simulink subsystem "processor"  (R2026a)
settings: Solver=VariableStepAuto
settings Model: Creator=finnb  LastModifiedBy=trist

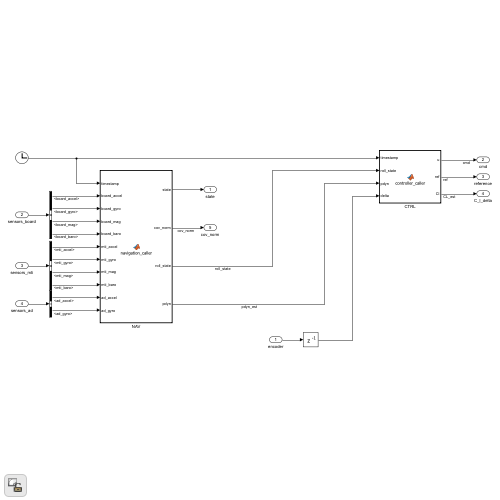
[thumbnail: Simulink's stored preview of the top-level diagram]
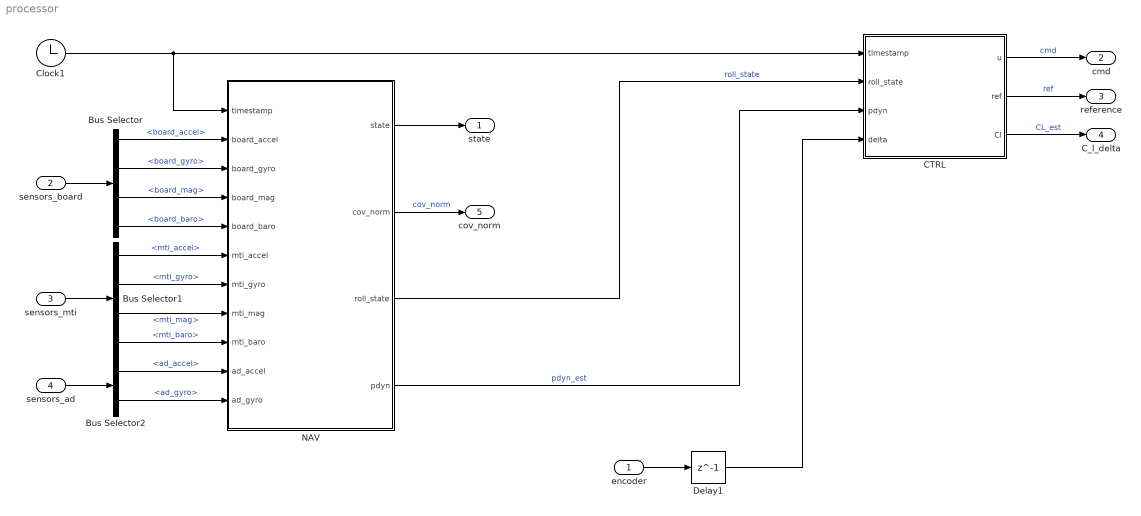
== system processor ==
  encoder : Inport
  sensors_board : Inport  Port=2
  sensors_mti : Inport  Port=3
  sensors_ad : Inport  Port=4
  Bus Selector : BusSelector  OutputSignals=board_accel,board_gyro,board_mag,board_baro
  Bus Selector1 : BusSelector  OutputSignals=mti_accel,mti_gyro,mti_mag,mti_baro
  Bus Selector2 : BusSelector  OutputSignals=ad_accel,ad_gyro
  CTRL : MATLAB Function  TreatAsAtomicUnit=on
  Clock1 : Clock
  Delay1 : Delay  DelayLength=1
  NAV : MATLAB Function  TreatAsAtomicUnit=on
  state : Outport
  cmd : Outport  Port=2
  reference : Outport  Port=3  PortDimensions=2
  C_l_delta : Outport  Port=4
  cov_norm : Outport  Port=5
  wires:
  Clock1/1 -> CTRL/1(timestamp), NAV/1(timestamp)
  NAV/1(state) -> state/1
  encoder/1 -> Delay1/1
  CTRL/1(u) -> cmd/1  "cmd"
  Delay1/1 -> CTRL/4(delta)
  CTRL/3(Cl) -> C_l_delta/1  "CL_est"
  sensors_board/1 -> Bus Selector/1
  sensors_mti/1 -> Bus Selector1/1
  sensors_ad/1 -> Bus Selector2/1
  Bus Selector/1 -> NAV/2(board_accel)  "<board_accel>"
  Bus Selector/2 -> NAV/3(board_gyro)  "<board_gyro>"
  Bus Selector/3 -> NAV/4(board_mag)  "<board_mag>"
  Bus Selector/4 -> NAV/5(board_baro)  "<board_baro>"
  Bus Selector1/1 -> NAV/6(mti_accel)  "<mti_accel>"
  Bus Selector1/2 -> NAV/7(mti_gyro)  "<mti_gyro>"
  Bus Selector1/3 -> NAV/8(mti_mag)  "<mti_mag>"
  Bus Selector1/4 -> NAV/9(mti_baro)  "<mti_baro>"
  Bus Selector2/2 -> NAV/11(ad_gyro)  "<ad_gyro>"
  Bus Selector2/1 -> NAV/10(ad_accel)  "<ad_accel>"
  NAV/2(cov_norm) -> cov_norm/1  "cov_norm"
  NAV/3(roll_state) -> CTRL/2(roll_state)  "roll_state"
  NAV/4(pdyn) -> CTRL/3(pdyn)  "pdyn_est"
  CTRL/2(ref) -> reference/1  "ref"

== matlab function processor/CTRL ==
  settings: updateMethod=DISCRETE  sampleTime=samplingtime_ctrl
  data: timestamp input size=1; roll_state input; pdyn input; delta input size=1; u output size=1; ref output; Cl output size=1
function [u, ref, Cl] = controller_caller(timestamp, roll_state, pdyn, delta)
    
    [u, ref, Cl] = controller_module(timestamp, roll_state, pdyn, delta);
 
end

== matlab function processor/NAV ==
  settings: updateMethod=DISCRETE  sampleTime=samplingtime_nav
  data: timestamp input size=1; board_accel input Bus: Sensor3DBus; board_gyro input Bus: Sensor3DBus; board_mag input Bus: Sensor3DBus; board_baro input Bus: Sensor1DBus; mti_accel input Bus: Sensor3DBus; mti_gyro input Bus: Sensor3DBus; mti_mag input Bus: Sensor3DBus; mti_baro input Bus: Sensor1DBus; ad_accel input Bus: Sensor3DBus; ad_gyro input Bus: Sensor3DBus; state output; cov_norm output; roll_state output; pdyn output
function [state, cov_norm, roll_state, pdyn] = navigation_caller(timestamp, board_accel, board_gyro, board_mag, board_baro, mti_accel, mti_gyro, mti_mag, mti_baro, ad_accel, ad_gyro)
    %#codegen

    %% IMU handler mock (rotation correction)
    board_accel.meas = sensor_handler(board_accel.meas, "board", "imu");
    board_gyro.meas = sensor_handler(board_gyro.meas, "board", "imu");
    mti_accel.meas = sensor_handler(mti_accel.meas, "mti", "imu");
    mti_gyro.meas = sensor_handler(mti_gyro.meas, "mti", "imu");
    ad_accel.meas = sensor_handler(ad_accel.meas, "ad", "imu");
    ad_gyro.meas = sensor_handler(ad_gyro.meas, "ad", "imu");
    board_mag.meas = sensor_handler(board_mag.meas, "board", "mag");
    mti_mag.meas = sensor_handler(mti_mag.meas, "mti", "mag");
    
    %%% baro does not need to be rotation corrected    

    %% Navigation
    state = zeros(11,1);
    cov_norm = 0;
    pdyn = 0;
    roll_state = [0; 0];
    [state, cov_norm, roll_state, pdyn] = navigation_module(timestamp, board_accel, board_gyro, mti_accel, mti_gyro, ad_accel, ad_gyro, board_baro, board_mag, mti_baro, mti_mag);  
end
